simulink model "LQR_comparison"  (Simulink 10.3)
settings: Solver=ode45  StartTime=0.0  StopTime=tsim  RelTol=1e-3  EnableMultiTasking=on
values from neighbouring files (symbols this model uses):
  A = [-1.2822 0 0.98 0; 0 0 1 0; -5.4293 0 -1.8366 0; -128.2 128.2 0 0]    [Razzo27.m]
  B = [-0.3 0 -17 0]'    [Razzo27.m]
  C = [0 1 0 0; 0 0 0 1; -128.2 128.2 0 0]    [Razzo27.m]
  C_states = eye(4)    [Razzo27.m]
  D_states = [0; 0; 0; 0]    [Razzo27.m]
  sat_max = deg2rad(15)    [Razzo27.m]
  sat_min = deg2rad(-15)    [Razzo27.m]
  x0 = [deg2rad(0) deg2rad(-15) 0 200]    [Razzo27.m]
  x_ref = [0 0 0 0]'    [Razzo27.m]
undefined symbols (not defined in the file or in its folder): Klqr1, Klqr2, Klqr3, Klqr4
settings Model: Creator=Administrator  LastModifiedBy=dadel  MultithreadedSim=on
settings DataIOCC: LimitDataPoints=on
settings OptimizationCC: InitFltsAndDblsToZero=on
settings ConfigComp: CovSFcnEnable=off

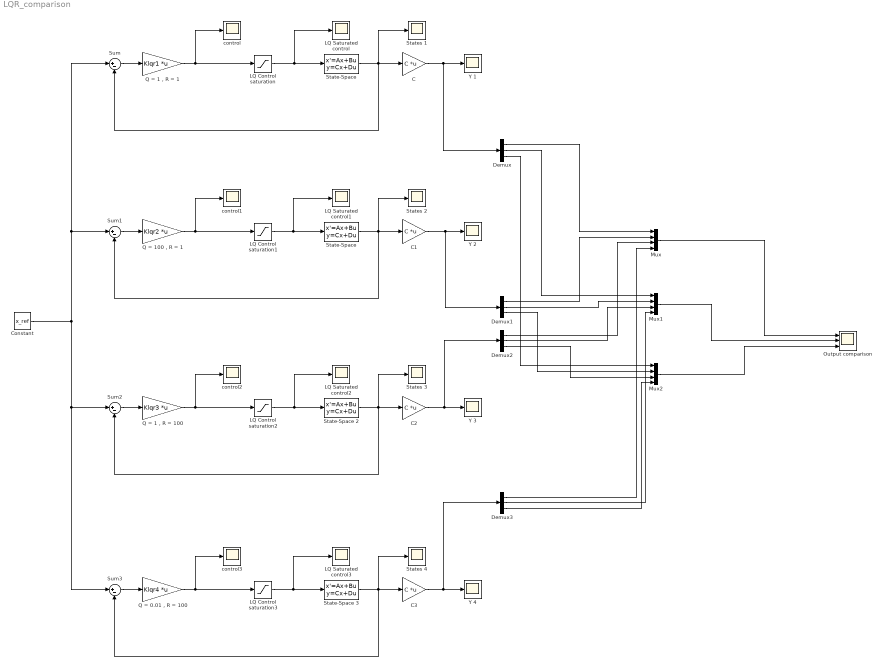
== system LQR_comparison ==
  C{,1..3} (4 alike) : Gain  Gain=C  Multiplication=Matrix(K*u)
  Constant : Constant  Value=x_ref
  Demux{,1..3} (4 alike) : Demux  Outputs=3
  LQ Control saturation{,1..3} (4 alike) : Saturate  UpperLimit=sat_max  LowerLimit=sat_min
  LQ Saturated control{,1..3} (4 alike) : Scope
  Mux : Mux
  Mux1 : Mux
  Mux2 : Mux
  "Output comparison  " : Scope  NumInputPorts=3
  "Q = 0.01 , R = 100" : Gain  Gain=Klqr4  Multiplication=Matrix(K*u)
  "Q = 1 , R = 1" : Gain  Gain=Klqr1  Multiplication=Matrix(K*u)
  "Q = 1 , R = 100" : Gain  Gain=Klqr3  Multiplication=Matrix(K*u)
  "Q = 100 , R = 1" : Gain  Gain=Klqr2  Multiplication=Matrix(K*u)
  State-Space : StateSpace  A=A  B=B  C=C_states  D=D_states  InitialCondition=x0
  "State-Space " : StateSpace  A=A  B=B  C=C_states  D=D_states  InitialCondition=x0
  State-Space 2 : StateSpace  A=A  B=B  C=C_states  D=D_states  InitialCondition=x0
  State-Space 3 : StateSpace  A=A  B=B  C=C_states  D=D_states  InitialCondition=x0
  States {1..4} (4 alike) : Scope
  Sum{,1..3} (4 alike) : Sum  Inputs=|+-
  Y {1..4} (4 alike) : Scope
  control{,1..3} (4 alike) : Scope
  wires:
  "Q = 1 , R = 1"/1 -> LQ Control saturation/1, control/1
  Sum/1 -> "Q = 1 , R = 1"/1
  "State-Space "/1 -> States 1/1, C/1, Sum/2
  Sum1/1 -> "Q = 100 , R = 1"/1
  C1/1 -> Y 2/1, Demux1/1
  "Q = 100 , R = 1"/1 -> LQ Control saturation1/1, control1/1
  State-Space/1 -> States 2/1, C1/1, Sum1/2
  Sum2/1 -> "Q = 1 , R = 100"/1
  C2/1 -> Y 3/1, Demux2/1
  "Q = 1 , R = 100"/1 -> LQ Control saturation2/1, control2/1
  State-Space 2/1 -> States 3/1, C2/1, Sum2/2
  Sum3/1 -> "Q = 0.01 , R = 100"/1
  C3/1 -> Y 4/1, Demux3/1
  "Q = 0.01 , R = 100"/1 -> LQ Control saturation3/1, control3/1
  State-Space 3/1 -> States 4/1, C3/1, Sum3/2
  C/1 -> Demux/1, Y 1/1
  Demux/1 -> Mux/1
  Demux1/1 -> Mux/2
  Demux2/1 -> Mux/3
  Demux3/1 -> Mux/4
  Demux1/2 -> Mux1/2
  Demux/2 -> Mux1/1
  Demux2/2 -> Mux1/3
  Demux3/2 -> Mux1/4
  Demux3/3 -> Mux2/4
  Demux2/3 -> Mux2/3
  Demux1/3 -> Mux2/2
  Demux/3 -> Mux2/1
  Mux/1 -> "Output comparison  "/1
  Mux1/1 -> "Output comparison  "/2
  Mux2/1 -> "Output comparison  "/3
  Constant/1 -> Sum1/1, Sum/1, Sum3/1, Sum2/1
  LQ Control saturation/1 -> LQ Saturated control/1, "State-Space "/1
  LQ Control saturation1/1 -> State-Space/1, LQ Saturated control1/1
  LQ Control saturation2/1 -> LQ Saturated control2/1, State-Space 2/1
  LQ Control saturation3/1 -> LQ Saturated control3/1, State-Space 3/1
